simulink model "EKF_slam_v4"  (R2021a)
settings: Solver=VariableStepAuto  StartTime=0.0  StopTime=P.SimTime  RelTol=1e-3
undefined symbols (not defined in the file or in its folder): drawvehicle4, Estimator_SLAML3, P, Sensor_model_v4
settings Model: Creator=sankepaa

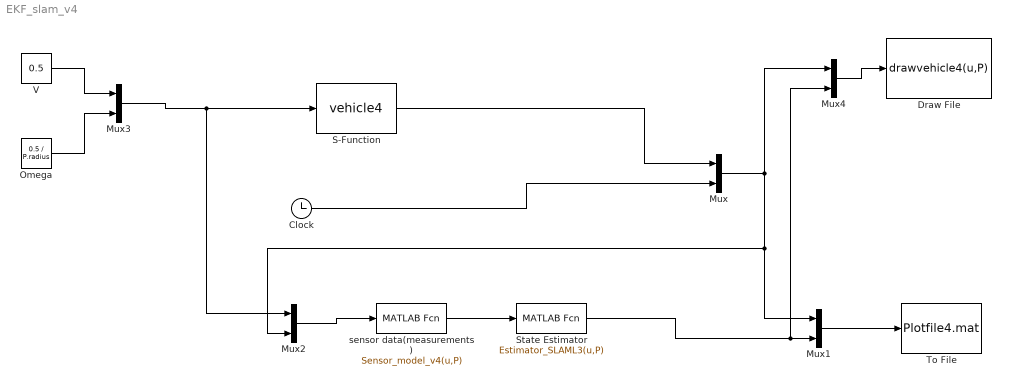
== system EKF_slam_v4 ==
  " sensor data(measurements) " : MATLABFcn  MATLABFcn=Sensor_model_v4(u,P)  OutputDimensions=3*P.NumLm + 2 + 1
  Clock : Clock
  "Draw File " : MATLABFcn  MATLABFcn=drawvehicle4(u,P)  OutputDimensions=0
  Mux{,1..4} (5 alike) : Mux  Inputs=2
  Omega : Constant  Value=0.5 / P.radius
  S-Function : S-Function  FunctionName=vehicle4  Parameters=P  SFunctionDeploymentMode=off  EnableBusSupport=off
  "State Estimator " : MATLABFcn  MATLABFcn=Estimator_SLAML3(u,P)  OutputDimensions=10
  To File : ToFile  Filename=Plotfile4.mat  MatrixName=dat  SaveFormat=Timeseries
  V : Constant  Value=0.5
  wires:
  S-Function/1 -> Mux/1
  " sensor data(measurements) "/1 -> "State Estimator "/1
  "State Estimator "/1 -> Mux4/2, Mux1/2
  Mux1/1 -> To File/1
  Clock/1 -> Mux/2
  Mux/1 -> Mux4/1, Mux2/2, Mux1/1
  V/1 -> Mux3/1
  Omega/1 -> Mux3/2
  Mux3/1 -> Mux2/1, S-Function/1
  Mux2/1 -> " sensor data(measurements) "/1
  Mux4/1 -> "Draw File "/1
